simulink model "dsppitchtime"  (Simulink 8.3)
settings: Solver=FixedStepDiscrete  StartTime=0.0  StopTime=4  RelTol=1e-3
PreLoadFcn:
  | load clean_speech.mat;
libraries: dspsigops x5, dspmtrx3 x4, dspxfrm3 x2, dspsnks4 x1, dspmisc x1, dspsrcs4 x1, dspswit3 x1
settings Model: Creator=The MathWorks Inc.  ExtModeAutoUpdateStatusClock=off
settings SolverCC: InsertRTBMode=Auto
settings DataIOCC: LimitDataPoints=off  SaveTime=off  OutputSaveName=y_pnt  SignalLoggingName=logsOut
settings OptimizationCC: InlineParams=on  InlineInvariantSignals=on  ExpressionDepthLimit=2147483647  InitFltsAndDblsToZero=on  EfficientMapNaN2IntZero=off
settings DebuggingCC: CheckExecutionContextPreStartOutputMsg=on  CheckExecutionContextRuntimeOutputMsg=on  SignalResolutionControl=TryResolveAllWithWarning  SolverPrmCheckMsg=none  MultiTaskDSMMsg=warning  MultiTaskCondExecSysMsg=none  FcnCallInpInsideContextMsg=UseLocalSettings
settings HardwareCC: ProdHWDeviceType=Specified
settings RTWCC: IncludeERTFirstTime=on
settings GRTTargetCC: TargetFcnLib=ansi_tfl_tmw_new.mat

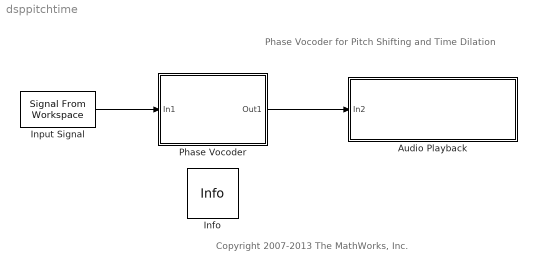
== system dsppitchtime ==
  note: Phase Vocoder for Pitch Shifting and Time Dilation
  note: Copyright 2007-2013 The MathWorks, Inc.
  Audio Playback : Subsystem  mask{effectType=Pitch Shifting}
      mask prompts: effectType "Type of effect:"
      mask TypeOptions effectType: Pitch Shifting | Time Dilation
      mask Callback effectType:
      | str = get_param('dsppitchtime/Audio Playback', 'effectType');
      | if strcmp(str, 'Pitch Shifting')
      |     set_param('dsppitchtime/Audio Playback/To Audio Device', 'InheritSampleRate','on');
      | else
      |     set_param('dsppitchtime/Audio Playback/To Audio Device', 'InheritSampleRate', 'off');
      | end
      mask DialogControl DescTextVar Prompt: Select the type of effect to be played on the audio output device
      mask Display:
      | str = get_param('dsppitchtime/Audio Playback', 'effectType');
      | disp(['Playback Mode: ', str, '\n', ...
      |     '[Double-click to change]']);
  Info : dspmisc/Info  SystemSampleTime=-1
  Input Signal : dspsrcs4/Signal From Workspace  X=Speech  Ts=1/8000  nsamps=64  OutputAfterFinalValue=Setting to zero  ignoreOrWarnInputAndFrameLengths=off
  Phase Vocoder : Subsystem  mask(Phase Vocoder){ana_hopSize=64, winLen=256, syn_hopSize=90}
      mask prompts: ana_hopSize "Analysis hop size (i.e., temporal shift of analysis window) (in samples):"; winLen "Window size (in samples):"; syn_hopSize "Synthesis hop size (i.e., temporal shift of synthesis window) (in samples):"
      mask help:
      | Algorithm for time dilation and pitch shifting of an audio signal. Time dilation changes the speed of an audio signal without affecting its pitch. Pitch shifting changes the pitch of an audio signal without affecting its speed.
      |
      | The pitch shifting and time dilation factors are defined by the ratio of the Synthesis hop size parameter to the Analysis hop size parameter.
      |
      | The Window size parameter must meet the following two requirements:
      | - log2(Window size) must be a positive integer
      | - Window size must be greater than both the Analysis hop size and the Synthesis hop size parameter values.
      mask Display: disp('Phase Vocoder')
  wires:
  Input Signal/1 -> Phase Vocoder/1(In1)
  Phase Vocoder/1(Out1) -> Audio Playback/1(In2)

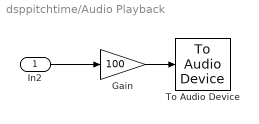
== system dsppitchtime/Audio Playback ==
  In2 : Inport
  Gain : Gain  Gain=100
  To Audio Device : dspsnks4/To Audio Device  deviceName=Default  inheritSampleRate=on  sampleRate=8000  deviceDatatype=Determine from input data type  autoBufferSize=on  bufferSize=4096  queueDuration=1  defaultOutputChannelMapping=on  outputChannelMapping=1:2
  wires:
  In2/1 -> Gain/1
  Gain/1 -> To Audio Device/1

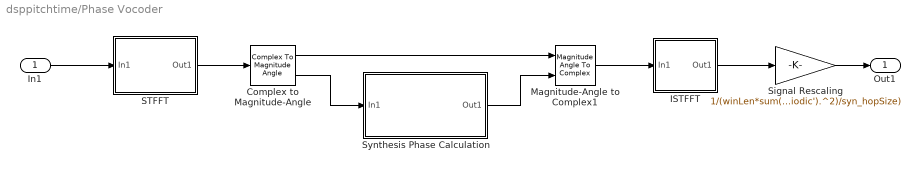
== system dsppitchtime/Phase Vocoder ==
  In1 : Inport
  Complex to Magnitude-Angle : ComplexToMagnitudeAngle
  ISTFFT : Subsystem
      mask Display: disp('Overlap\nIST-FFT')
  Magnitude-Angle to Complex1 : MagnitudeAngleToComplex
  STFFT : Subsystem
      mask Display: disp('Overlap\nST-FFT')
  Signal Rescaling : Gain  Gain=1/(winLen*sum(hanning(winLen,'periodic').^2)/syn_hopSize)  OutDataTypeStr=Inherit: Same as input  ParamDataTypeStr=Inherit: Same as input
  Synthesis Phase Calculation : Subsystem  mask{ana_hopSize=ana_hopSize, syn_hopSize=syn_hopSize, winLen=winLen}
      mask prompts: ana_hopSize "Analysis hop size:"; syn_hopSize "Synthesis hop size:"; winLen "Window size:"
      mask Display: disp('Synthesis\nPhase\nCalculation')
  Out1 : Outport
  wires:
  In1/1 -> STFFT/1(In1)
  STFFT/1(Out1) -> Complex to Magnitude-Angle/1
  Magnitude-Angle to Complex1/1 -> ISTFFT/1(In1)
  ISTFFT/1(Out1) -> Signal Rescaling/1
  Complex to Magnitude-Angle/2 -> Synthesis Phase Calculation/1(In1)
  Complex to Magnitude-Angle/1 -> Magnitude-Angle to Complex1/1
  Synthesis Phase Calculation/1(Out1) -> Magnitude-Angle to Complex1/2
  Signal Rescaling/1 -> Out1/1

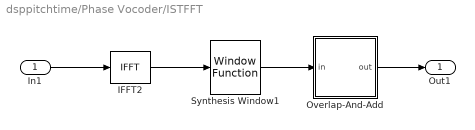
== system dsppitchtime/Phase Vocoder/ISTFFT ==
  In1 : Inport
  IFFT2 : dspxfrm3/IFFT  CompMethod=Table lookup  TableOpt=HYBRID  TableOptActive=Speed  BitRevOrder=off  cs_in=on  SkipNorm=on  InheritFFTLength=on  FFTLength=64  WrapInput=on  mode=Complex  outSamplingMode=Frame based  RowConvenienceOn=on  FFTImplementation=Auto  firstCoeffMode=User-defined  firstCoeffWordLength=16  firstCoeffFracLength=15  firstCoeffDataTypeStr=fixdt(1,16)  firstCoeffLastDataTypeStr=fixdt(1,16)  outputMin=[]  outputMax=[]  accumDataTypeStr=Inherit: Same as product output  accumLastDataTypeStr=Inherit: Same as product output  roundingMode=Floor  overflowMode=off
  Overlap-And-Add : Subsystem  mask(Overlap-And-Add){L=syn_hopSize}
      mask prompts: L "Number of new points in each frame"
      mask help: Performs overlap-and-add on the input signal. Disjoint frames of the input signal are overlapped with each other for a specified number of points and summed.
      mask Display: disp('Overlap\nAnd\nAdd')
  Synthesis Window1 : dspsigops/Window Function  winmode=Apply window to input  wintype=Hanning  sampmode=Continuous  samptime=1  N=64  Rs=50  beta=10  winsamp=Periodic  UserWindow=hamming  OptParams=off  UserParams={1.0}  RowConvenienceOn=on  dataType=double  isSigned=on  wordLen=16  udDataType=sfix(16)  fracBitsMode=Best precision  numFracBits=15  roundingMode=Floor  overflowMode=off  numSidelobes=4  sidelobeLevel=-30
  Out1 : Outport
  wires:
  IFFT2/1 -> Synthesis Window1/1
  Overlap-And-Add/1(out) -> Out1/1
  In1/1 -> IFFT2/1
  Synthesis Window1/1 -> Overlap-And-Add/1(in)

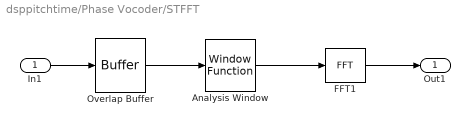
== system dsppitchtime/Phase Vocoder/STFFT ==
  In1 : Inport
  Analysis Window : dspsigops/Window Function  winmode=Apply window to input  wintype=Hanning  sampmode=Continuous  samptime=1  N=64  Rs=50  beta=10  winsamp=Periodic  UserWindow=hamming  OptParams=off  UserParams={1.0}  RowConvenienceOn=on  dataType=double  isSigned=on  wordLen=16  udDataType=sfix(16)  fracBitsMode=Best precision  numFracBits=15  roundingMode=Floor  overflowMode=off  numSidelobes=4  sidelobeLevel=-30
  FFT1 : dspxfrm3/FFT  CompMethod=Table lookup  TableOpt=NEW  TableOptActive=Speed  BitRevOrder=off  InheritFFTLength=on  FFTLength=64  WrapInput=on  RowConvenienceOn=on  FFTImplementation=Auto  SkipNorm=off  firstCoeffMode=Specify word length  firstCoeffWordLength=16  firstCoeffFracLength=15  firstCoeffDataTypeStr=fixdt(1,16)  firstCoeffLastDataTypeStr=fixdt(1,16)  outputMin=[]  outputMax=[]  accumDataTypeStr=Inherit: Same as product output  accumLastDataTypeStr=Inherit: Same as product output  roundingMode=Floor  overflowMode=off
  Overlap Buffer : Buffer  N=winLen  V=winLen-ana_hopSize  TreatMby1Signals=One channel
  Out1 : Outport
  wires:
  Overlap Buffer/1 -> Analysis Window/1
  FFT1/1 -> Out1/1
  In1/1 -> Overlap Buffer/1
  Analysis Window/1 -> FFT1/1

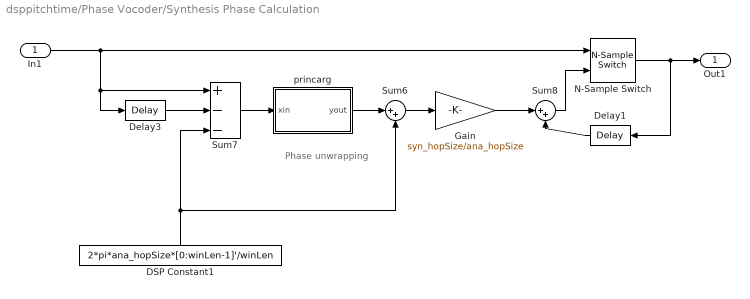
== system dsppitchtime/Phase Vocoder/Synthesis Phase Calculation ==
  note: Phase unwrapping
  In1 : Inport
  DSP Constant1 : Constant  Value=2*pi*ana_hopSize*[0:winLen-1]'/winLen  VectorParams1D=off  SampleTime=64/8000
  Delay1 : dspsigops/Delay  dly_unit=Frames  delay=1  ic_detail=on  dif_ic_for_ch=off  dif_ic_for_dly=off  ic=0  reset_popup=None
  Delay3 : dspsigops/Delay  dly_unit=Frames  delay=1  ic_detail=on  dif_ic_for_ch=off  dif_ic_for_dly=off  ic=0  reset_popup=None
  Gain : Gain  Gain=syn_hopSize/ana_hopSize  OutDataTypeStr=Inherit: Same as input  ParamDataTypeStr=Inherit: Same as input
  N-Sample Switch : dspswit3/N-Sample Switch  N=1  reset=off  TriggerType=Rising edge  Ts=-1
  Sum6 : Sum  Inputs=|++  SaturateOnIntegerOverflow=on
  Sum7 : Sum  Inputs=+--  SaturateOnIntegerOverflow=on
  Sum8 : Sum  Inputs=|++  SaturateOnIntegerOverflow=on
  princarg : Subsystem
      mask Display: disp('Principal\nArgument');
  Out1 : Outport
  wires:
  In1/1 -> N-Sample Switch/1, Delay3/1, Sum7/1
  Delay3/1 -> Sum7/2
  DSP Constant1/1 -> Sum7/3, Sum6/2
  Sum7/1 -> princarg/1(xin)
  princarg/1(yout) -> Sum6/1
  Sum6/1 -> Gain/1
  Gain/1 -> Sum8/1
  N-Sample Switch/1 -> Delay1/1, Out1/1
  Delay1/1 -> Sum8/2
  Sum8/1 -> N-Sample Switch/2

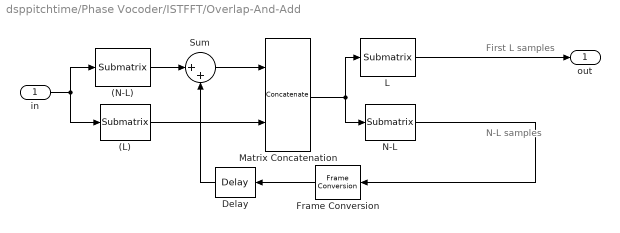
== system dsppitchtime/Phase Vocoder/ISTFFT/Overlap-And-Add ==
  note: First L samples
  note: N-L samples
  in : Inport
  (L) : dspmtrx3/Submatrix  RowSpan=Range of rows  RowStartMode=Offset from last  RowStartIndex=L-1  RowEndMode=Last  RowEndIndex=1  ColSpan=All columns  ColStartMode=First  ColStartIndex=1  ColEndMode=Last  ColEndIndex=1
  (N-L) : dspmtrx3/Submatrix  RowSpan=Range of rows  RowStartMode=First  RowStartIndex=1  RowEndMode=Offset from last  RowEndIndex=L  ColSpan=All columns  ColStartMode=First  ColStartIndex=1  ColEndMode=Last  ColEndIndex=1
  Delay : dspsigops/Delay  dly_unit=Samples  delay=1  ic_detail=off  dif_ic_for_ch=off  dif_ic_for_dly=off  ic=0  reset_popup=None
  Frame Conversion : FrameConversion  OutFrame=Sample-based
  L : dspmtrx3/Submatrix  RowSpan=Range of rows  RowStartMode=First  RowStartIndex=1  RowEndMode=Index  RowEndIndex=L  ColSpan=All columns  ColStartMode=First  ColStartIndex=1  ColEndMode=Last  ColEndIndex=1
  Matrix Concatenation : Concatenate  Mode=Multidimensional array
  N-L : dspmtrx3/Submatrix  RowSpan=Range of rows  RowStartMode=Index  RowStartIndex=L+1  RowEndMode=Last  RowEndIndex=1  ColSpan=All columns  ColStartMode=First  ColStartIndex=1  ColEndMode=Last  ColEndIndex=1
  Sum : Sum  Inputs=|++  SaturateOnIntegerOverflow=on  InputSameDT=on  OutDataTypeStr=Inherit: Same as first input
  out : Outport
  wires:
  L/1 -> out/1
  Sum/1 -> Matrix Concatenation/1
  (N-L)/1 -> Sum/1
  Delay/1 -> Sum/2
  (L)/1 -> Matrix Concatenation/2
  N-L/1 -> Frame Conversion/1
  Matrix Concatenation/1 -> L/1, N-L/1
  in/1 -> (L)/1, (N-L)/1
  Frame Conversion/1 -> Delay/1

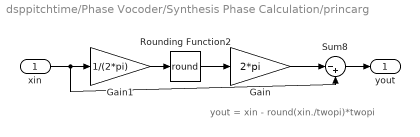
== system dsppitchtime/Phase Vocoder/Synthesis Phase Calculation/princarg ==
  note: yout = xin - round(xin./twopi)*twopi
  xin : Inport
  Gain : Gain  Gain=2*pi  OutDataTypeStr=Inherit: Same as input  ParamDataTypeStr=Inherit: Same as input
  Gain1 : Gain  Gain=1/(2*pi)  OutDataTypeStr=Inherit: Same as input  ParamDataTypeStr=Inherit: Same as input
  Rounding Function2 : Rounding  Operator=round
  Sum8 : Sum  Inputs=|-+  SaturateOnIntegerOverflow=on
  yout : Outport
  wires:
  xin/1 -> Sum8/2, Gain1/1
  Gain1/1 -> Rounding Function2/1
  Rounding Function2/1 -> Gain/1
  Gain/1 -> Sum8/1
  Sum8/1 -> yout/1
